simulink model "mytopologybat"  (R2014b)
settings: Solver=ode23tb  StartTime=0.0  StopTime=1  MaxStep=0.0001  MinStep=0.00001  RelTol=1e-3
libraries: powerlib x130, simulink x45, powerlib_meascontrol x2
(part 2 of 2)

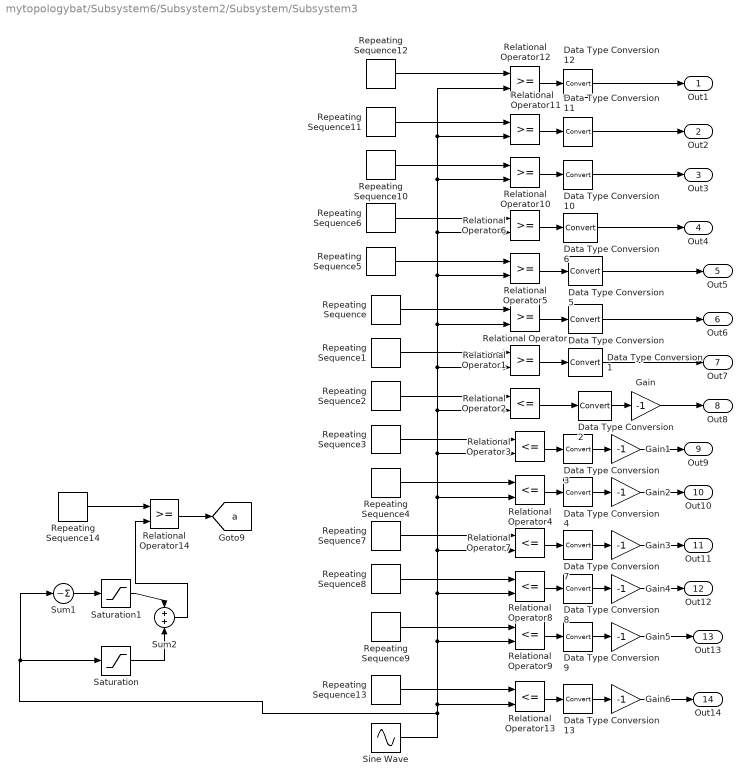
== system mytopologybat/Subsystem6/Subsystem2/Subsystem/Subsystem3 ==
  Data Type Conversion{,1..13} (14 alike) : DataTypeConversion
  Gain{,1..6} (7 alike) : Gain  Gain=-1
  Relational Operator{,1,5..6,10..12,14} (8 alike) : RelationalOperator  OutDataTypeStr=boolean
  Relational Operator{2..4,7..9,13} (7 alike) : RelationalOperator  Operator=<=  OutDataTypeStr=boolean
  Repeating Sequence : simulink/Sources/Repeating Sequence  rep_seq_t="[0 (1/fc)/2  (1/fc)]"  rep_seq_y=[1 2 1]
  Repeating Sequence1 : simulink/Sources/Repeating Sequence  rep_seq_t="[0 (1/fc)/2  (1/fc)]"  rep_seq_y=[0 1 0]
  Repeating Sequence10 : simulink/Sources/Repeating Sequence  rep_seq_t="[0 (1/fc)/2  (1/fc)]"  rep_seq_y=[4 5 4]
  Repeating Sequence11 : simulink/Sources/Repeating Sequence  rep_seq_t="[0 (1/fc)/2  (1/fc)]"  rep_seq_y=[5 6 5]
  Repeating Sequence12 : simulink/Sources/Repeating Sequence  rep_seq_t="[0 (1/fc)/2  (1/fc)]"  rep_seq_y=[6 7 6]
  Repeating Sequence13 : simulink/Sources/Repeating Sequence  rep_seq_t="[0 (1/fc)/2  (1/fc)]"  rep_seq_y=[-7 -6 -7]
  Repeating Sequence14 : simulink/Sources/Repeating Sequence  rep_seq_t="[0 (1/fc)/2  (1/fc)]"  rep_seq_y=[0 1 0]
  Repeating Sequence2 : simulink/Sources/Repeating Sequence  rep_seq_t="[0 (1/fc)/2  (1/fc)]"  rep_seq_y=[-1 0 -1]
  Repeating Sequence3 : simulink/Sources/Repeating Sequence  rep_seq_t="[0 (1/fc)/2  (1/fc)]"  rep_seq_y=[-2 -1 -2]
  Repeating Sequence4 : simulink/Sources/Repeating Sequence  rep_seq_t="[0 (1/fc)/2  (1/fc)]"  rep_seq_y=[-3 -2 -3]
  Repeating Sequence5 : simulink/Sources/Repeating Sequence  rep_seq_t="[0 (1/fc)/2  (1/fc)]"  rep_seq_y=[2 3 2]
  Repeating Sequence6 : simulink/Sources/Repeating Sequence  rep_seq_t="[0 (1/fc)/2  (1/fc)]"  rep_seq_y=[3 4 3]
  Repeating Sequence7 : simulink/Sources/Repeating Sequence  rep_seq_t="[0 (1/fc)/2  (1/fc)]"  rep_seq_y=[-4 -3 -4]
  Repeating Sequence8 : simulink/Sources/Repeating Sequence  rep_seq_t="[0 (1/fc)/2  (1/fc)]"  rep_seq_y=[-5 -4 -5]
  Repeating Sequence9 : simulink/Sources/Repeating Sequence  rep_seq_t="[0 (1/fc)/2  (1/fc)]"  rep_seq_y=[-6 -5 -6]
  Saturation : Saturate  UpperLimit=1  LowerLimit=0
  Saturation1 : Saturate  UpperLimit=1  LowerLimit=0
  Sine Wave : Sin  Amplitude=7*m  Frequency=2*pi*50  SampleTime=0
  Sum1 : Sum  Inputs=-
  Sum2 : Sum
  Out1 : Outport
  Out2 : Outport  Port=2
  Out3 : Outport  Port=3
  Out4 : Outport  Port=4
  Out5 : Outport  Port=5
  Out6 : Outport  Port=6
  Out7 : Outport  Port=7
  Out8 : Outport  Port=8
  Out9 : Outport  Port=9
  Out10 : Outport  Port=10
  Out11 : Outport  Port=11
  Out12 : Outport  Port=12
  Out13 : Outport  Port=13
  Out14 : Outport  Port=14
  tag scope: a=global
  wires:
  Relational Operator/1 -> Data Type Conversion/1
  Relational Operator1/1 -> Data Type Conversion1/1
  Repeating Sequence/1 -> Relational Operator/1
  Repeating Sequence1/1 -> Relational Operator1/1
  Repeating Sequence2/1 -> Relational Operator2/1
  Repeating Sequence3/1 -> Relational Operator3/1
  Relational Operator2/1 -> Data Type Conversion2/1
  Relational Operator3/1 -> Data Type Conversion3/1
  Data Type Conversion2/1 -> Gain/1
  Data Type Conversion3/1 -> Gain1/1
  Repeating Sequence4/1 -> Relational Operator4/1
  Relational Operator4/1 -> Data Type Conversion4/1
  Data Type Conversion4/1 -> Gain2/1
  Relational Operator5/1 -> Data Type Conversion5/1
  Repeating Sequence5/1 -> Relational Operator5/1
  Relational Operator6/1 -> Data Type Conversion6/1
  Repeating Sequence6/1 -> Relational Operator6/1
  Repeating Sequence7/1 -> Relational Operator7/1
  Relational Operator7/1 -> Data Type Conversion7/1
  Data Type Conversion7/1 -> Gain3/1
  Repeating Sequence8/1 -> Relational Operator8/1
  Relational Operator8/1 -> Data Type Conversion8/1
  Data Type Conversion8/1 -> Gain4/1
  Repeating Sequence9/1 -> Relational Operator9/1
  Relational Operator9/1 -> Data Type Conversion9/1
  Data Type Conversion9/1 -> Gain5/1
  Repeating Sequence10/1 -> Relational Operator10/1
  Relational Operator10/1 -> Data Type Conversion10/1
  Repeating Sequence11/1 -> Relational Operator11/1
  Relational Operator11/1 -> Data Type Conversion11/1
  Relational Operator12/1 -> Data Type Conversion12/1
  Repeating Sequence12/1 -> Relational Operator12/1
  Repeating Sequence13/1 -> Relational Operator13/1
  Relational Operator13/1 -> Data Type Conversion13/1
  Data Type Conversion13/1 -> Gain6/1
  Data Type Conversion12/1 -> Out1/1
  Data Type Conversion11/1 -> Out2/1
  Data Type Conversion10/1 -> Out3/1
  Data Type Conversion6/1 -> Out4/1
  Data Type Conversion5/1 -> Out5/1
  Data Type Conversion/1 -> Out6/1
  Data Type Conversion1/1 -> Out7/1
  Gain/1 -> Out8/1
  Gain1/1 -> Out9/1
  Gain2/1 -> Out10/1
  Gain3/1 -> Out11/1
  Gain4/1 -> Out12/1
  Gain5/1 -> Out13/1
  Gain6/1 -> Out14/1
  Sine Wave/1 -> Sum1/1, Saturation/1, Relational Operator13/2, Relational Operator9/2, Relational Operator8/2, Relational Operator7/2, Relational Operator4/2, Relational Operator3/2, Relational Operator2/2, Relational Operator1/2, Relational Operator/2, Relational Operator5/2, Relational Operator6/2, Relational Operator10/2, Relational Operator11/2, Relational Operator12/2
  Sum1/1 -> Saturation1/1
  Saturation1/1 -> Sum2/1
  Saturation/1 -> Sum2/2
  Repeating Sequence14/1 -> Relational Operator14/1
  Sum2/1 -> Relational Operator14/2
  Relational Operator14/1 -> [a]

== system mytopologybat/Subsystem6/Subsystem3/Subsystem2/If Action Subsystem ==
  In1 : Inport
  Action Port : ActionPort  ActionType=case
  Out1 : Outport
  wires:
  In1/1 -> Out1/1

== system mytopologybat/Subsystem6/Subsystem3/Subsystem2/If Action Subsystem1 ==
  In1 : Inport
  Action Port : ActionPort  ActionType=case
  Out1 : Outport
  wires:
  In1/1 -> Out1/1

== system mytopologybat/Subsystem6/Subsystem3/Subsystem2/If Action Subsystem10 ==
  In1 : Inport
  Action Port : ActionPort  ActionType=case
  Out1 : Outport
  wires:
  In1/1 -> Out1/1

== system mytopologybat/Subsystem6/Subsystem3/Subsystem2/If Action Subsystem11 ==
  In1 : Inport
  Action Port : ActionPort  ActionType=case
  Out1 : Outport
  wires:
  In1/1 -> Out1/1

== system mytopologybat/Subsystem6/Subsystem3/Subsystem2/If Action Subsystem12 ==
  In1 : Inport
  Action Port : ActionPort  ActionType=case
  Out1 : Outport
  wires:
  In1/1 -> Out1/1

== system mytopologybat/Subsystem6/Subsystem3/Subsystem2/If Action Subsystem13 ==
  In1 : Inport
  Action Port : ActionPort  ActionType=case
  Out1 : Outport
  wires:
  In1/1 -> Out1/1

== system mytopologybat/Subsystem6/Subsystem3/Subsystem2/If Action Subsystem14 ==
  In1 : Inport
  Action Port : ActionPort  ActionType=case
  Out1 : Outport
  wires:
  In1/1 -> Out1/1

== system mytopologybat/Subsystem6/Subsystem3/Subsystem2/If Action Subsystem2 ==
  In1 : Inport
  Action Port : ActionPort  ActionType=case
  Out1 : Outport
  wires:
  In1/1 -> Out1/1

== system mytopologybat/Subsystem6/Subsystem3/Subsystem2/If Action Subsystem3 ==
  In1 : Inport
  Action Port : ActionPort  ActionType=case
  Out1 : Outport
  wires:
  In1/1 -> Out1/1

== system mytopologybat/Subsystem6/Subsystem3/Subsystem2/If Action Subsystem4 ==
  In1 : Inport
  Action Port : ActionPort  ActionType=case
  Out1 : Outport
  wires:
  In1/1 -> Out1/1

== system mytopologybat/Subsystem6/Subsystem3/Subsystem2/If Action Subsystem5 ==
  In1 : Inport
  Action Port : ActionPort  ActionType=case
  Out1 : Outport
  wires:
  In1/1 -> Out1/1

== system mytopologybat/Subsystem6/Subsystem3/Subsystem2/If Action Subsystem6 ==
  In1 : Inport
  Action Port : ActionPort  ActionType=case
  Out1 : Outport
  wires:
  In1/1 -> Out1/1

== system mytopologybat/Subsystem6/Subsystem3/Subsystem2/If Action Subsystem7 ==
  In1 : Inport
  Action Port : ActionPort  ActionType=case
  Out1 : Outport
  wires:
  In1/1 -> Out1/1

== system mytopologybat/Subsystem6/Subsystem3/Subsystem2/If Action Subsystem8 ==
  In1 : Inport
  Action Port : ActionPort  ActionType=case
  Out1 : Outport
  wires:
  In1/1 -> Out1/1

== system mytopologybat/Subsystem6/Subsystem3/Subsystem2/If Action Subsystem9 ==
  In1 : Inport
  Action Port : ActionPort  ActionType=case
  Out1 : Outport
  wires:
  In1/1 -> Out1/1

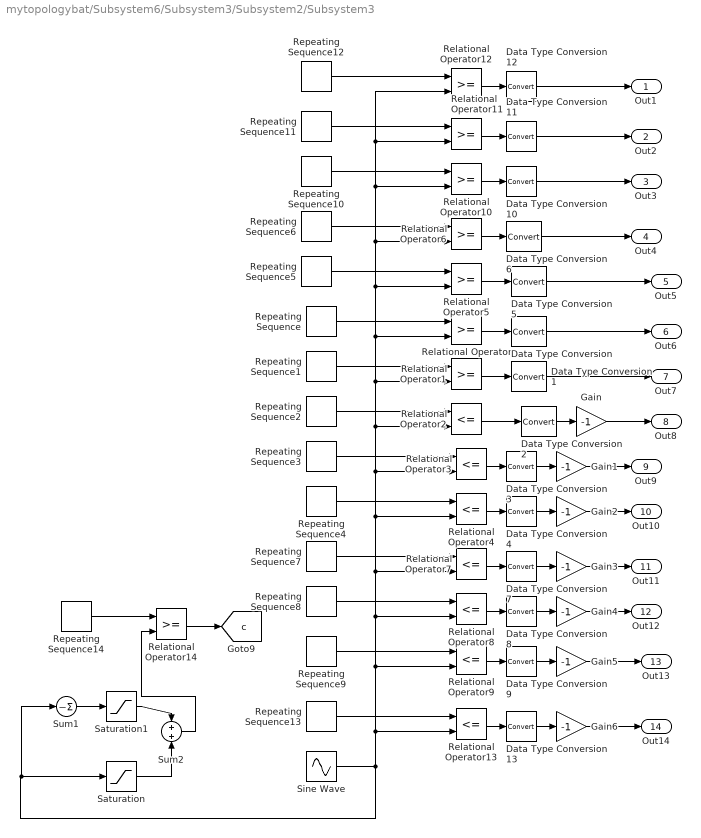
== system mytopologybat/Subsystem6/Subsystem3/Subsystem2/Subsystem3 ==
  Data Type Conversion{,1..13} (14 alike) : DataTypeConversion
  Gain{,1..6} (7 alike) : Gain  Gain=-1
  Relational Operator{,1,5..6,10..12,14} (8 alike) : RelationalOperator  OutDataTypeStr=boolean
  Relational Operator{2..4,7..9,13} (7 alike) : RelationalOperator  Operator=<=  OutDataTypeStr=boolean
  Repeating Sequence : simulink/Sources/Repeating Sequence  rep_seq_t="[0 (1/fc)/2  (1/fc)]"  rep_seq_y=[1 2 1]
  Repeating Sequence1 : simulink/Sources/Repeating Sequence  rep_seq_t="[0 (1/fc)/2  (1/fc)]"  rep_seq_y=[0 1 0]
  Repeating Sequence10 : simulink/Sources/Repeating Sequence  rep_seq_t="[0 (1/fc)/2  (1/fc)]"  rep_seq_y=[4 5 4]
  Repeating Sequence11 : simulink/Sources/Repeating Sequence  rep_seq_t="[0 (1/fc)/2  (1/fc)]"  rep_seq_y=[5 6 5]
  Repeating Sequence12 : simulink/Sources/Repeating Sequence  rep_seq_t="[0 (1/fc)/2  (1/fc)]"  rep_seq_y=[6 7 6]
  Repeating Sequence13 : simulink/Sources/Repeating Sequence  rep_seq_t="[0 (1/fc)/2  (1/fc)]"  rep_seq_y=[-7 -6 -7]
  Repeating Sequence14 : simulink/Sources/Repeating Sequence  rep_seq_t="[0 (1/fc)/2  (1/fc)]"  rep_seq_y=[0 1 0]
  Repeating Sequence2 : simulink/Sources/Repeating Sequence  rep_seq_t="[0 (1/fc)/2  (1/fc)]"  rep_seq_y=[-1 0 -1]
  Repeating Sequence3 : simulink/Sources/Repeating Sequence  rep_seq_t="[0 (1/fc)/2  (1/fc)]"  rep_seq_y=[-2 -1 -2]
  Repeating Sequence4 : simulink/Sources/Repeating Sequence  rep_seq_t="[0 (1/fc)/2  (1/fc)]"  rep_seq_y=[-3 -2 -3]
  Repeating Sequence5 : simulink/Sources/Repeating Sequence  rep_seq_t="[0 (1/fc)/2  (1/fc)]"  rep_seq_y=[2 3 2]
  Repeating Sequence6 : simulink/Sources/Repeating Sequence  rep_seq_t="[0 (1/fc)/2  (1/fc)]"  rep_seq_y=[3 4 3]
  Repeating Sequence7 : simulink/Sources/Repeating Sequence  rep_seq_t="[0 (1/fc)/2  (1/fc)]"  rep_seq_y=[-4 -3 -4]
  Repeating Sequence8 : simulink/Sources/Repeating Sequence  rep_seq_t="[0 (1/fc)/2  (1/fc)]"  rep_seq_y=[-5 -4 -5]
  Repeating Sequence9 : simulink/Sources/Repeating Sequence  rep_seq_t="[0 (1/fc)/2  (1/fc)]"  rep_seq_y=[-6 -5 -6]
  Saturation : Saturate  UpperLimit=10  LowerLimit=0
  Saturation1 : Saturate  UpperLimit=10  LowerLimit=0
  Sine Wave : Sin  Amplitude=7*m  Frequency=2*pi*50  Phase=-2*pi/3  SampleTime=0
  Sum1 : Sum  Inputs=-
  Sum2 : Sum
  Out1 : Outport
  Out2 : Outport  Port=2
  Out3 : Outport  Port=3
  Out4 : Outport  Port=4
  Out5 : Outport  Port=5
  Out6 : Outport  Port=6
  Out7 : Outport  Port=7
  Out8 : Outport  Port=8
  Out9 : Outport  Port=9
  Out10 : Outport  Port=10
  Out11 : Outport  Port=11
  Out12 : Outport  Port=12
  Out13 : Outport  Port=13
  Out14 : Outport  Port=14
  tag scope: c=global
  wires:
  Relational Operator/1 -> Data Type Conversion/1
  Relational Operator1/1 -> Data Type Conversion1/1
  Repeating Sequence/1 -> Relational Operator/1
  Repeating Sequence1/1 -> Relational Operator1/1
  Repeating Sequence2/1 -> Relational Operator2/1
  Repeating Sequence3/1 -> Relational Operator3/1
  Relational Operator2/1 -> Data Type Conversion2/1
  Relational Operator3/1 -> Data Type Conversion3/1
  Data Type Conversion2/1 -> Gain/1
  Data Type Conversion3/1 -> Gain1/1
  Repeating Sequence4/1 -> Relational Operator4/1
  Relational Operator4/1 -> Data Type Conversion4/1
  Data Type Conversion4/1 -> Gain2/1
  Relational Operator5/1 -> Data Type Conversion5/1
  Repeating Sequence5/1 -> Relational Operator5/1
  Relational Operator6/1 -> Data Type Conversion6/1
  Repeating Sequence6/1 -> Relational Operator6/1
  Repeating Sequence7/1 -> Relational Operator7/1
  Relational Operator7/1 -> Data Type Conversion7/1
  Data Type Conversion7/1 -> Gain3/1
  Repeating Sequence8/1 -> Relational Operator8/1
  Relational Operator8/1 -> Data Type Conversion8/1
  Data Type Conversion8/1 -> Gain4/1
  Repeating Sequence9/1 -> Relational Operator9/1
  Relational Operator9/1 -> Data Type Conversion9/1
  Data Type Conversion9/1 -> Gain5/1
  Repeating Sequence10/1 -> Relational Operator10/1
  Relational Operator10/1 -> Data Type Conversion10/1
  Repeating Sequence11/1 -> Relational Operator11/1
  Relational Operator11/1 -> Data Type Conversion11/1
  Relational Operator12/1 -> Data Type Conversion12/1
  Repeating Sequence12/1 -> Relational Operator12/1
  Repeating Sequence13/1 -> Relational Operator13/1
  Relational Operator13/1 -> Data Type Conversion13/1
  Data Type Conversion13/1 -> Gain6/1
  Data Type Conversion12/1 -> Out1/1
  Data Type Conversion11/1 -> Out2/1
  Data Type Conversion10/1 -> Out3/1
  Data Type Conversion6/1 -> Out4/1
  Data Type Conversion5/1 -> Out5/1
  Data Type Conversion/1 -> Out6/1
  Data Type Conversion1/1 -> Out7/1
  Gain/1 -> Out8/1
  Gain1/1 -> Out9/1
  Gain2/1 -> Out10/1
  Gain3/1 -> Out11/1
  Gain4/1 -> Out12/1
  Gain5/1 -> Out13/1
  Gain6/1 -> Out14/1
  Relational Operator14/1 -> [c]
  Sum2/1 -> Relational Operator14/2
  Repeating Sequence14/1 -> Relational Operator14/1
  Saturation/1 -> Sum2/2
  Saturation1/1 -> Sum2/1
  Sum1/1 -> Saturation1/1
  Sine Wave/1 -> Relational Operator13/2, Relational Operator9/2, Relational Operator8/2, Relational Operator7/2, Relational Operator4/2, Relational Operator3/2, Relational Operator2/2, Relational Operator1/2, Relational Operator/2, Relational Operator5/2, Relational Operator6/2, Relational Operator10/2, Relational Operator11/2, Relational Operator12/2, Saturation/1, Sum1/1
